simulink subsystem "desacople_realimentacion_fisicas_naturales"  (R2023b)
settings: Solver=VariableStepAuto  StartTime=0.0  StopTime=10.0  RelTol=1e-3
values from neighbouring files (symbols this model uses):
  L_d = 6.6    [main.m]    (also in parametros.m = 0.0066)
  L_q = 5.8e-3    (= 0.0058)    [diagrama_polos_y_ceros_LTI.m]    (also in main.m = 5.8; parametros.m; variacion_de_parametros.m)
  lambda_m = 0.016    [main.m]    (also in parametros.m)
  P_p = 3    [diagrama_polos_y_ceros_LTI.m]    (also in main.m; parametros.m; variacion_de_parametros.m)
settings Model: Creator=nicol  LastModifiedBy=nicol

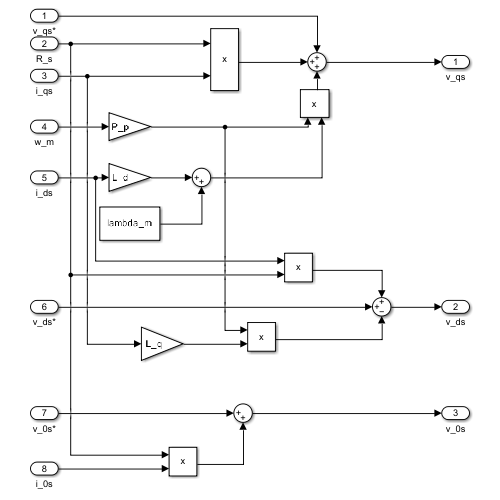
[thumbnail: Simulink's stored preview of the top-level diagram]
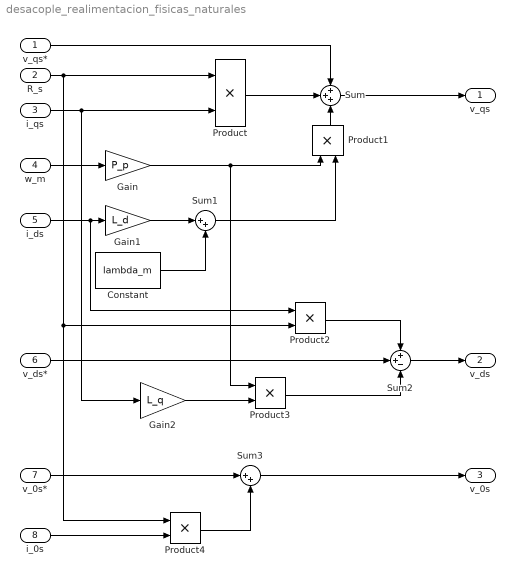
== system desacople_realimentacion_fisicas_naturales ==
  v_qs* : Inport
  R_s : Inport  Port=2
  i_qs : Inport  Port=3
  w_m : Inport  Port=4
  i_ds : Inport  Port=5
  v_ds* : Inport  Port=6
  v_0s* : Inport  Port=7
  i_0s : Inport  Port=8
  Constant : Constant  Value=lambda_m
  Gain : Gain  Gain=P_p
  Gain1 : Gain  Gain=L_d
  Gain2 : Gain  Gain=L_q
  Product{,1..4} (5 alike) : Product
  Sum : Sum  Inputs=+++
  Sum1 : Sum  Inputs=|++
  Sum2 : Sum  Inputs=++-
  Sum3 : Sum  Inputs=|++
  v_qs : Outport
  v_ds : Outport  Port=2
  v_0s : Outport  Port=3
  wires:
  i_qs/1 -> Gain2/1, Product/2
  R_s/1 -> Product2/2, Product4/1, Product/1
  v_qs*/1 -> Sum/1
  Product/1 -> Sum/2
  Sum/1 -> v_qs/1
  Product1/1 -> Sum/3
  Gain/1 -> Product3/1, Product1/1
  Constant/1 -> Sum1/2
  Gain1/1 -> Sum1/1
  i_ds/1 -> Product2/1, Gain1/1
  w_m/1 -> Gain/1
  Sum1/1 -> Product1/2
  Sum2/1 -> v_ds/1
  v_ds*/1 -> Sum2/2
  Product2/1 -> Sum2/1
  Gain2/1 -> Product3/2
  Product3/1 -> Sum2/3
  v_0s*/1 -> Sum3/1
  i_0s/1 -> Product4/2
  Product4/1 -> Sum3/2
  Sum3/1 -> v_0s/1
